simulink model "SVPWM_closeloop"  (R2022a)
settings: Solver=ode23t  StartTime=0.0  StopTime=1  RelTol=1e-3
InitFcn:
  | disp('开关频率20000Hz')
  | Ts = 1/20000;
libraries: spsIGBTDiodeLib x12, spsSeriesRLCBranchLib x11, spsDiodeLib x6, slpidlib x5, spsVoltageMeasurementLib x4, spsabctodq0Lib x3, spsThreePhaseVIMeasurementLib x2, spsDCVoltageSourceLib x1, spsGroundLib x1, spsPower3phInstantaneousLib x1, simulink x1, spsdq0toabcLib x1
settings Model: Creator=Ziang Liu  LastModifiedBy=Ziang Liu
settings DataIOCC: ReturnWorkspaceOutputs=off

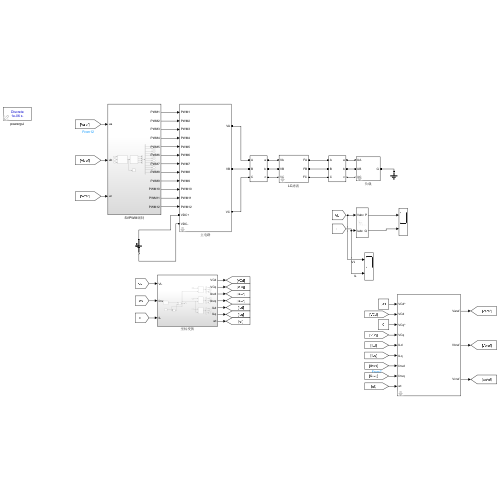
[thumbnail: Simulink's stored preview of the top-level diagram]
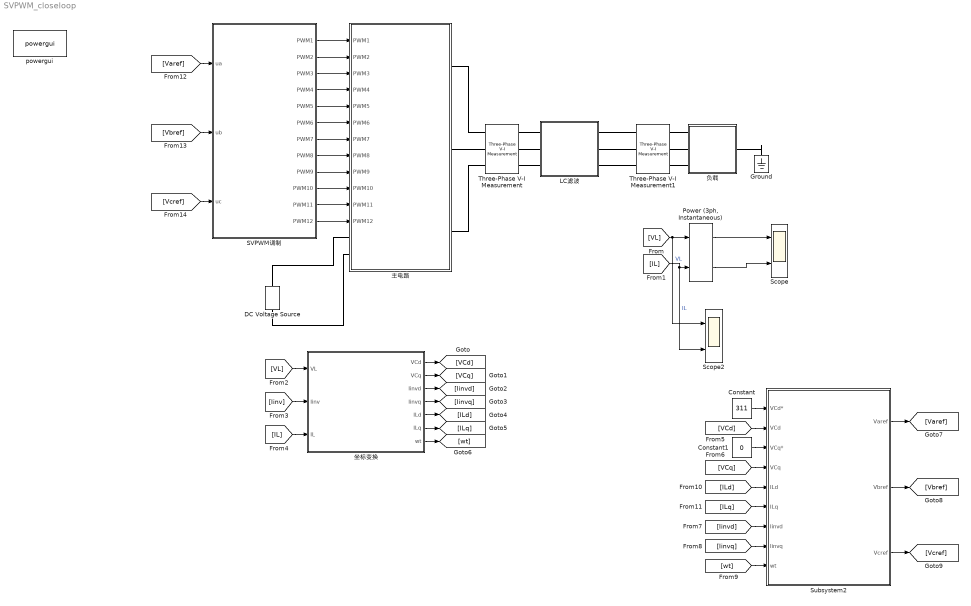
== system SVPWM_closeloop ==
  Constant : Constant  Value=311
  Constant1 : Constant  Value=0
  DC Voltage Source : spsDCVoltageSourceLib/DC Voltage Source  Amplitude=800  Measurements=None
  Ground : spsGroundLib/Ground  LConnTagsString=a
  LC滤波 : Subsystem  mask{L0=2e-3, R0=1e-3, Cf=10.5e-6, RC=3}
      mask prompts: L0 "滤波电感L0："; R0 "寄生电阻R0"; Cf "滤波电容Cf："; RC "无源阻尼RC："
      mask DialogControl ParameterGroupVar Prompt: 参数
  "Power (3ph, Instantaneous)" : spsPower3phInstantaneousLib/Power (3ph, Instantaneous)
  SVPWM调制 : Subsystem
  Scope : Scope  NumInputPorts=2
  Scope2 : Scope  NumInputPorts=2
  Subsystem2 : Subsystem  mask{Kp1=1.0825, Ki1=27.59, Kp2=13.3, Ki2=6.67, wC=2*pi*50*10.5e-6, wL=2*pi*50*2e-3}
      mask prompts: Kp1 "电压外环Kp1"; Ki1 "电压外环Ki1"; Kp2 "电流内环Kp2"; Ki2 "电流内环Ki2"; wC "电容耦合wC"; wL "电感耦合wL"
      mask DialogControl ParameterGroupVar Prompt: 参数
  Three-Phase V-I Measurement : spsThreePhaseVIMeasurementLib/Three-Phase V-I Measurement  VoltageMeasurement=no  SetLabelV=off  LabelV=Vabc  Vpu=off  VpuLL=off  CurrentMeasurement=yes  SetLabelI=on  LabelI=Iinv  Ipu=off  Pbase=100e6  Vbase=500e3  OutputType=Complex  PhasorSimulation=off  PSBequivalent=0
  Three-Phase V-I Measurement1 : spsThreePhaseVIMeasurementLib/Three-Phase V-I Measurement  VoltageMeasurement=phase-to-ground  SetLabelV=on  LabelV=VL  Vpu=off  VpuLL=off  CurrentMeasurement=yes  SetLabelI=on  LabelI=IL  Ipu=off  Pbase=100e6  Vbase=500e3  OutputType=Complex  PhasorSimulation=off  PSBequivalent=0
  powergui : spspowerguiLib/powergui  Priority=1  SimulationMode=Discrete  SampleTime=1e-6  frequency=60  Iterations=50  frequencyindice=0  Pbase=100e6  ErrMax=1e-4  UnitsV=kV  UnitsW=MW  buscounter=0  FunctionMessages=off  echomessages=off  EnableUseOfTLC=off  CurrentSourceSwitches=off  DisableSnubberDevices=off  DisableRonSwitches=off  DisableVfSwitches=off  DisplayEquations=off  AutomaticDiscreteSolvers=off  SolverType=Tustin/Backward Euler (TBE)  Interpol=off  ExternalGateDelay=off  methode=off  Ts=100  x0status=blocks  SPID=on  SwTol=0  HookPort=off  NonlinearTolerance=1e-4  nMaxIteration=100  ContinueOnMaxIteration=off  RestoreLinks=warning  ResistiveCurrentMeasurement=off  Frange=[0:2:500]  Ylog=off  Xlog=on  ShowGrid=off  save=off  variable=ZData  structure=0  ZoomFFT=off  StartTime=0.0  cycles=1  DisplayStyle=1  fundamental=60  FreqAxis=off  MaxFrequency=1000  frequencyindicesteady=1  RmsSteady=1  display=off
  主电路 : Subsystem  mask{C0=5600e-6}
      mask prompts: C0 "直流电容C0:"
      mask DialogControl ParameterGroupVar Prompt: 参数
  坐标变换 : Subsystem
  负载 : Subsystem  mask{R=1.44, L=0, C=3e-3}
      mask prompts: R "负载电阻R"; L "负载电感L"; C "负载电容C"
      mask DialogControl ParameterGroupVar Prompt: 参数
  wires:
  [Varef] -> SVPWM调制/1(ua)
  [Vbref] -> SVPWM调制/2(ub)
  [Vcref] -> SVPWM调制/3(uc)
  SVPWM调制/1(PWM1) -> 主电路/1(PWM1)
  SVPWM调制/2(PWM2) -> 主电路/2(PWM2)
  SVPWM调制/3(PWM3) -> 主电路/3(PWM3)
  SVPWM调制/4(PWM4) -> 主电路/4(PWM4)
  SVPWM调制/5(PWM5) -> 主电路/5(PWM5)
  SVPWM调制/6(PWM6) -> 主电路/6(PWM6)
  SVPWM调制/7(PWM7) -> 主电路/7(PWM7)
  SVPWM调制/8(PWM8) -> 主电路/8(PWM8)
  SVPWM调制/9(PWM9) -> 主电路/9(PWM9)
  SVPWM调制/10(PWM10) -> 主电路/10(PWM10)
  SVPWM调制/11(PWM11) -> 主电路/11(PWM11)
  SVPWM调制/12(PWM12) -> 主电路/12(PWM12)
  [VL] -> Scope2/1, "Power (3ph, Instantaneous)"/1  "VL"
  [IL] -> Scope2/2, "Power (3ph, Instantaneous)"/2  "IL"
  "Power (3ph, Instantaneous)"/1 -> Scope/1
  "Power (3ph, Instantaneous)"/2 -> Scope/2
  [Iinv] -> 坐标变换/2(Iinv)
  [VL] -> 坐标变换/1(VL)
  [IL] -> 坐标变换/3(IL)
  坐标变换/1(VCd) -> [VCd]
  坐标变换/2(VCq) -> [VCq]
  坐标变换/3(Iinvd) -> [Iinvd]
  坐标变换/4(Iinvq) -> [Iinvq]
  坐标变换/5(ILd) -> [ILd]
  坐标变换/6(ILq) -> [ILq]
  坐标变换/7(wt) -> [wt]
  Constant/1 -> Subsystem2/1(VCd*)
  Constant1/1 -> Subsystem2/3(VCq*)
  [VCd] -> Subsystem2/2(VCd)
  [VCq] -> Subsystem2/4(VCq)
  [Iinvd] -> Subsystem2/7(Iinvd)
  [Iinvq] -> Subsystem2/8(Iinvq)
  [wt] -> Subsystem2/9(wt)
  [ILd] -> Subsystem2/5(ILd)
  [ILq] -> Subsystem2/6(ILq)
  Subsystem2/1(Varef) -> [Varef]
  Subsystem2/2(Vbref) -> [Vbref]
  Subsystem2/3(Vcref) -> [Vcref]
  connections:
  DC Voltage Source/RConn1 -- 主电路/LConn1
  DC Voltage Source/LConn1 -- 主电路/LConn2
  Three-Phase V-I Measurement/LConn2 -- 主电路/RConn2
  主电路/RConn1 -- Three-Phase V-I Measurement/LConn1
  主电路/RConn3 -- Three-Phase V-I Measurement/LConn3
  LC滤波/LConn1 -- Three-Phase V-I Measurement/RConn1
  LC滤波/LConn2 -- Three-Phase V-I Measurement/RConn2
  LC滤波/LConn3 -- Three-Phase V-I Measurement/RConn3
  Three-Phase V-I Measurement1/LConn1 -- LC滤波/RConn1
  Three-Phase V-I Measurement1/LConn2 -- LC滤波/RConn2
  Three-Phase V-I Measurement1/LConn3 -- LC滤波/RConn3
  负载/LConn1 -- Three-Phase V-I Measurement1/RConn1
  负载/LConn2 -- Three-Phase V-I Measurement1/RConn2
  负载/LConn3 -- Three-Phase V-I Measurement1/RConn3
  Ground/LConn1 -- 负载/RConn1

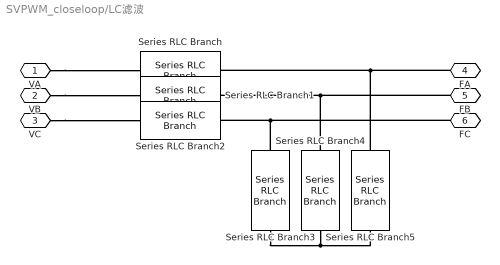
== system SVPWM_closeloop/LC滤波 ==
  Series RLC Branch : spsSeriesRLCBranchLib/Series RLC Branch  LConnTagsString=__new0  RConnTagsString=__new0  BranchType=RL  Resistance=R0  Inductance=L0  SetiL0=off  InitialCurrent=0  Capacitance=1e-6  Setx0=off  InitialVoltage=0  Measurements=None
  Series RLC Branch1 : spsSeriesRLCBranchLib/Series RLC Branch  LConnTagsString=__new0  RConnTagsString=__new0  BranchType=RL  Resistance=R0  Inductance=L0  SetiL0=off  InitialCurrent=0  Capacitance=1e-6  Setx0=off  InitialVoltage=0  Measurements=None
  Series RLC Branch2 : spsSeriesRLCBranchLib/Series RLC Branch  LConnTagsString=__new0  RConnTagsString=__new0  BranchType=RL  Resistance=R0  Inductance=L0  SetiL0=off  InitialCurrent=0  Capacitance=1e-6  Setx0=off  InitialVoltage=0  Measurements=None
  Series RLC Branch3 : spsSeriesRLCBranchLib/Series RLC Branch  LConnTagsString=__new0  RConnTagsString=__new0  BranchType=RC  Resistance=RC  Inductance=L0  SetiL0=off  InitialCurrent=0  Capacitance=Cf  Setx0=off  InitialVoltage=0  Measurements=None
  Series RLC Branch4 : spsSeriesRLCBranchLib/Series RLC Branch  LConnTagsString=__new0  RConnTagsString=__new0  BranchType=RC  Resistance=RC  Inductance=L0  SetiL0=off  InitialCurrent=0  Capacitance=Cf  Setx0=off  InitialVoltage=0  Measurements=None
  Series RLC Branch5 : spsSeriesRLCBranchLib/Series RLC Branch  LConnTagsString=__new0  RConnTagsString=__new0  BranchType=RC  Resistance=RC  Inductance=L0  SetiL0=off  InitialCurrent=0  Capacitance=Cf  Setx0=off  InitialVoltage=0  Measurements=None
  VA : PMIOPort  Side=Left
  VB : PMIOPort  Port=2  Side=Left
  VC : PMIOPort  Port=3  Side=Left
  FA : PMIOPort  Port=4  Side=Right
  FB : PMIOPort  Port=5  Side=Right
  FC : PMIOPort  Port=6  Side=Right
  connections:
  Series RLC Branch3/LConn1 -- FC/RConn1 -- Series RLC Branch2/RConn1
  Series RLC Branch4/LConn1 -- FB/RConn1 -- Series RLC Branch1/RConn1
  Series RLC Branch3/RConn1 -- Series RLC Branch4/RConn1 -- Series RLC Branch5/RConn1
  Series RLC Branch5/LConn1 -- FA/RConn1 -- Series RLC Branch/RConn1
  VB/RConn1 -- Series RLC Branch1/LConn1
  VA/RConn1 -- Series RLC Branch/LConn1
  VC/RConn1 -- Series RLC Branch2/LConn1

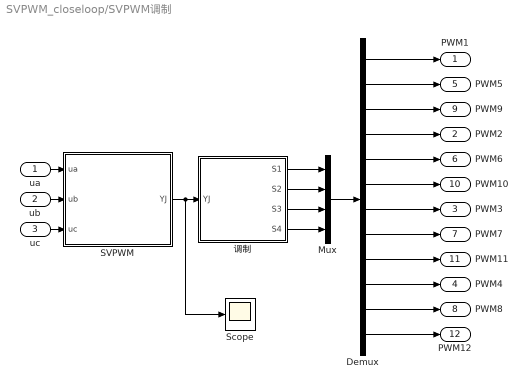
== system SVPWM_closeloop/SVPWM调制 ==
  ua : Inport
  ub : Inport  Port=2
  uc : Inport  Port=3
  Demux : Demux  Outputs=12
  Mux : Mux
  SVPWM : Subsystem
  Scope : Scope
  调制 : Subsystem
  PWM1 : Outport
  PWM2 : Outport  Port=2
  PWM3 : Outport  Port=3
  PWM4 : Outport  Port=4
  PWM5 : Outport  Port=5
  PWM6 : Outport  Port=6
  PWM7 : Outport  Port=7
  PWM8 : Outport  Port=8
  PWM9 : Outport  Port=9
  PWM10 : Outport  Port=10
  PWM11 : Outport  Port=11
  PWM12 : Outport  Port=12
  wires:
  Demux/4 -> PWM2/1
  Demux/9 -> PWM11/1
  SVPWM/1(YJ) -> Scope/1, 调制/1(YJ)
  ub/1 -> SVPWM/2(ub)
  Mux/1 -> Demux/1
  Demux/10 -> PWM4/1
  Demux/2 -> PWM5/1
  Demux/1 -> PWM1/1
  Demux/3 -> PWM9/1
  Demux/8 -> PWM7/1
  ua/1 -> SVPWM/1(ua)
  Demux/11 -> PWM8/1
  Demux/5 -> PWM6/1
  调制/4(S4) -> Mux/4
  调制/1(S1) -> Mux/1
  Demux/6 -> PWM10/1
  Demux/12 -> PWM12/1
  uc/1 -> SVPWM/3(uc)
  调制/3(S3) -> Mux/3
  调制/2(S2) -> Mux/2
  Demux/7 -> PWM3/1

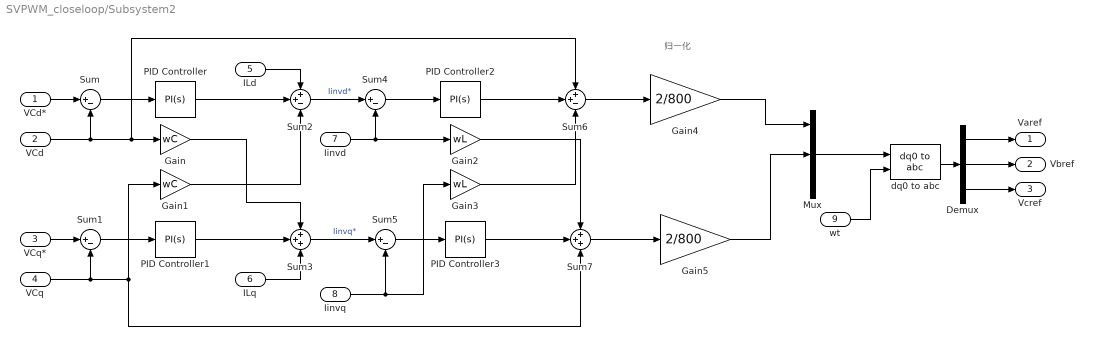
== system SVPWM_closeloop/Subsystem2 ==
  note: 归一化
  VCd* : Inport
  VCd : Inport  Port=2
  VCq* : Inport  Port=3
  VCq : Inport  Port=4
  ILd : Inport  Port=5
  ILq : Inport  Port=6
  Iinvd : Inport  Port=7
  Iinvq : Inport  Port=8
  wt : Inport  Port=9
  Demux : Demux  Outputs=3
  Gain : Gain  Gain=wC
  Gain1 : Gain  Gain=wC
  Gain2 : Gain  Gain=wL
  Gain3 : Gain  Gain=wL
  Gain4 : Gain  Gain=2/800
  Gain5 : Gain  Gain=2/800
  Mux : Mux  Inputs=3
  PID Controller : slpidlib/PID Controller  Controller=PI  Form=Parallel  TimeDomain=Continuous-time  UseExternalTs=off  SampleTime=-1  IntegratorMethod=Forward Euler  FilterMethod=Forward Euler  ControllerParametersSource=internal  P=Kp1  I=Ki1  UseKiTs=off  D=0  N=100  UseFilter=on  TunerSelectOption=Transfer Function Based (PID Tuner App)  InitialConditionSource=internal  InitialConditionForIntegrator=0  InitialConditionForFilter=0  DifferentiatorICPrevScaledInput=0  ExternalReset=none  TrackingMode=off  Kt=1  LimitOutput=off  SatLimitsSource=internal  UpperSaturationLimit=inf  LowerSaturationLimit=-inf  LinearizeAsGain=on  AntiWindupMode=none  Kb=1  POutMin=[]  POutMax=[]  IOutMin=[]  IOutMax=[]  DOutMin=[]  DOutMax=[]  NOutMin=[]  NOutMax=[]  SumOutMin=[]  SumOutMax=[]  SaturationOutMin=[]  SaturationOutMax=[]  PParamMin=[]  PParamMax=[]  IParamMin=[]  IParamMax=[]  DParamMin=[]  DParamMax=[]  NParamMin=[]  NParamMax=[]  KbParamMin=[]  KbParamMax=[]  KtParamMin=[]  KtParamMax=[]  KbOutMin=[]  KbOutMax=[]  KtOutMin=[]  KtOutMax=[]  IntegratorOutMin=[]  IntegratorOutMax=[]  FilterOutMin=[]  FilterOutMax=[]  SumI1OutMin=[]  SumI1OutMax=[]  SumI2OutMin=[]  SumI2OutMax=[]  SumI3OutMin=[]  SumI3OutMax=[]  SumI4OutMin=[]  SumI4OutMax=[]  SumDOutMin=[]  SumDOutMax=[]  DifferentiatorOutMin=[]  DifferentiatorOutMax=[]  FilterDiffOutCoefMin=[]  FilterDiffOutCoefMax=[]  ReciprocalOutMin=[]  ReciprocalOutMax=[]  SumDenOutMin=[]  SumDenOutMax=[]  SumNumOutMin=[]  SumNumOutMax=[]  DivideOutMin=[]  DivideOutMax=[]  UdiffTsProdOutMin=[]  UdiffTsProdOutMax=[]  NTsProdOutMin=[]  NTsProdOutMax=[]  UintegralTsProdOutMin=[]  UintegralTsProdOutMax=[]  UngainTsProdOutMin=[]  UngainTsProdOutMax=[]  IntegratorContinuousStateAttributes=''  IntegratorStateMustResolveToSignalObject=off  IntegratorRTWStateStorageClass=Auto  FilterContinuousStateAttributes=''  FilterStateMustResolveToSignalObject=off  FilterRTWStateStorageClass=Auto  ParallelPVariant=InternalParameters  IdealPVariant=Disabled  IVariant=InternalParameters  DVariant=Disabled  IntegratorVariant=Continuous  SatVariant=Disabled  AWVariant=Passthrough  PCopyVariant=Disabled  TRVariant=Disabled  FdbkBlocksVariant=Forward  IdealPFdbkVariant=Disabled  SatFdbkVariant=Disabled  DerivativeFilterVariant=Disabled  NVariant=Disabled  NCopyVariant=Disabled_SignalSpec  FilterICVariant=Disabled  IntegratorICVariant=InternalICs  ExternalResetVariant=Disabled  TRSumVariant=Passthrough  SumFdbkVariant=Disabled  SumVariant=Sum_PI  TsampFilterVariant=InternalTs  TsampNgainVariant=Passthrough  TsampIntegralVariant=Passthrough  ExternalSaturationOutDataTypeStr=Inherit: Same as second input  aMode=0
  PID Controller1 : slpidlib/PID Controller  Controller=PI  Form=Parallel  TimeDomain=Continuous-time  UseExternalTs=off  SampleTime=-1  IntegratorMethod=Forward Euler  FilterMethod=Forward Euler  ControllerParametersSource=internal  P=Kp1  I=Ki1  UseKiTs=off  D=0  N=100  UseFilter=on  TunerSelectOption=Transfer Function Based (PID Tuner App)  InitialConditionSource=internal  InitialConditionForIntegrator=0  InitialConditionForFilter=0  DifferentiatorICPrevScaledInput=0  ExternalReset=none  TrackingMode=off  Kt=1  LimitOutput=off  SatLimitsSource=internal  UpperSaturationLimit=inf  LowerSaturationLimit=-inf  LinearizeAsGain=on  AntiWindupMode=none  Kb=1  POutMin=[]  POutMax=[]  IOutMin=[]  IOutMax=[]  DOutMin=[]  DOutMax=[]  NOutMin=[]  NOutMax=[]  SumOutMin=[]  SumOutMax=[]  SaturationOutMin=[]  SaturationOutMax=[]  PParamMin=[]  PParamMax=[]  IParamMin=[]  IParamMax=[]  DParamMin=[]  DParamMax=[]  NParamMin=[]  NParamMax=[]  KbParamMin=[]  KbParamMax=[]  KtParamMin=[]  KtParamMax=[]  KbOutMin=[]  KbOutMax=[]  KtOutMin=[]  KtOutMax=[]  IntegratorOutMin=[]  IntegratorOutMax=[]  FilterOutMin=[]  FilterOutMax=[]  SumI1OutMin=[]  SumI1OutMax=[]  SumI2OutMin=[]  SumI2OutMax=[]  SumI3OutMin=[]  SumI3OutMax=[]  SumI4OutMin=[]  SumI4OutMax=[]  SumDOutMin=[]  SumDOutMax=[]  DifferentiatorOutMin=[]  DifferentiatorOutMax=[]  FilterDiffOutCoefMin=[]  FilterDiffOutCoefMax=[]  ReciprocalOutMin=[]  ReciprocalOutMax=[]  SumDenOutMin=[]  SumDenOutMax=[]  SumNumOutMin=[]  SumNumOutMax=[]  DivideOutMin=[]  DivideOutMax=[]  UdiffTsProdOutMin=[]  UdiffTsProdOutMax=[]  NTsProdOutMin=[]  NTsProdOutMax=[]  UintegralTsProdOutMin=[]  UintegralTsProdOutMax=[]  UngainTsProdOutMin=[]  UngainTsProdOutMax=[]  IntegratorContinuousStateAttributes=''  IntegratorStateMustResolveToSignalObject=off  IntegratorRTWStateStorageClass=Auto  FilterContinuousStateAttributes=''  FilterStateMustResolveToSignalObject=off  FilterRTWStateStorageClass=Auto  ParallelPVariant=InternalParameters  IdealPVariant=Disabled  IVariant=InternalParameters  DVariant=Disabled  IntegratorVariant=Continuous  SatVariant=Disabled  AWVariant=Passthrough  PCopyVariant=Disabled  TRVariant=Disabled  FdbkBlocksVariant=Forward  IdealPFdbkVariant=Disabled  SatFdbkVariant=Disabled  DerivativeFilterVariant=Disabled  NVariant=Disabled  NCopyVariant=Disabled_SignalSpec  FilterICVariant=Disabled  IntegratorICVariant=InternalICs  ExternalResetVariant=Disabled  TRSumVariant=Passthrough  SumFdbkVariant=Disabled  SumVariant=Sum_PI  TsampFilterVariant=InternalTs  TsampNgainVariant=Passthrough  TsampIntegralVariant=Passthrough  ExternalSaturationOutDataTypeStr=Inherit: Same as second input  aMode=0
  PID Controller2 : slpidlib/PID Controller  Controller=PI  Form=Parallel  TimeDomain=Continuous-time  UseExternalTs=off  SampleTime=-1  IntegratorMethod=Forward Euler  FilterMethod=Forward Euler  ControllerParametersSource=internal  P=Kp2  I=Ki2  UseKiTs=off  D=0  N=100  UseFilter=on  TunerSelectOption=Transfer Function Based (PID Tuner App)  InitialConditionSource=internal  InitialConditionForIntegrator=0  InitialConditionForFilter=0  DifferentiatorICPrevScaledInput=0  ExternalReset=none  TrackingMode=off  Kt=1  LimitOutput=off  SatLimitsSource=internal  UpperSaturationLimit=inf  LowerSaturationLimit=-inf  LinearizeAsGain=on  AntiWindupMode=none  Kb=1  POutMin=[]  POutMax=[]  IOutMin=[]  IOutMax=[]  DOutMin=[]  DOutMax=[]  NOutMin=[]  NOutMax=[]  SumOutMin=[]  SumOutMax=[]  SaturationOutMin=[]  SaturationOutMax=[]  PParamMin=[]  PParamMax=[]  IParamMin=[]  IParamMax=[]  DParamMin=[]  DParamMax=[]  NParamMin=[]  NParamMax=[]  KbParamMin=[]  KbParamMax=[]  KtParamMin=[]  KtParamMax=[]  KbOutMin=[]  KbOutMax=[]  KtOutMin=[]  KtOutMax=[]  IntegratorOutMin=[]  IntegratorOutMax=[]  FilterOutMin=[]  FilterOutMax=[]  SumI1OutMin=[]  SumI1OutMax=[]  SumI2OutMin=[]  SumI2OutMax=[]  SumI3OutMin=[]  SumI3OutMax=[]  SumI4OutMin=[]  SumI4OutMax=[]  SumDOutMin=[]  SumDOutMax=[]  DifferentiatorOutMin=[]  DifferentiatorOutMax=[]  FilterDiffOutCoefMin=[]  FilterDiffOutCoefMax=[]  ReciprocalOutMin=[]  ReciprocalOutMax=[]  SumDenOutMin=[]  SumDenOutMax=[]  SumNumOutMin=[]  SumNumOutMax=[]  DivideOutMin=[]  DivideOutMax=[]  UdiffTsProdOutMin=[]  UdiffTsProdOutMax=[]  NTsProdOutMin=[]  NTsProdOutMax=[]  UintegralTsProdOutMin=[]  UintegralTsProdOutMax=[]  UngainTsProdOutMin=[]  UngainTsProdOutMax=[]  IntegratorContinuousStateAttributes=''  IntegratorStateMustResolveToSignalObject=off  IntegratorRTWStateStorageClass=Auto  FilterContinuousStateAttributes=''  FilterStateMustResolveToSignalObject=off  FilterRTWStateStorageClass=Auto  ParallelPVariant=InternalParameters  IdealPVariant=Disabled  IVariant=InternalParameters  DVariant=Disabled  IntegratorVariant=Continuous  SatVariant=Disabled  AWVariant=Passthrough  PCopyVariant=Disabled  TRVariant=Disabled  FdbkBlocksVariant=Forward  IdealPFdbkVariant=Disabled  SatFdbkVariant=Disabled  DerivativeFilterVariant=Disabled  NVariant=Disabled  NCopyVariant=Disabled_SignalSpec  FilterICVariant=Disabled  IntegratorICVariant=InternalICs  ExternalResetVariant=Disabled  TRSumVariant=Passthrough  SumFdbkVariant=Disabled  SumVariant=Sum_PI  TsampFilterVariant=InternalTs  TsampNgainVariant=Passthrough  TsampIntegralVariant=Passthrough  ExternalSaturationOutDataTypeStr=Inherit: Same as second input  aMode=0
  PID Controller3 : slpidlib/PID Controller  Controller=PI  Form=Parallel  TimeDomain=Continuous-time  UseExternalTs=off  SampleTime=-1  IntegratorMethod=Forward Euler  FilterMethod=Forward Euler  ControllerParametersSource=internal  P=Kp2  I=Ki2  UseKiTs=off  D=0  N=100  UseFilter=on  TunerSelectOption=Transfer Function Based (PID Tuner App)  InitialConditionSource=internal  InitialConditionForIntegrator=0  InitialConditionForFilter=0  DifferentiatorICPrevScaledInput=0  ExternalReset=none  TrackingMode=off  Kt=1  LimitOutput=off  SatLimitsSource=internal  UpperSaturationLimit=inf  LowerSaturationLimit=-inf  LinearizeAsGain=on  AntiWindupMode=none  Kb=1  POutMin=[]  POutMax=[]  IOutMin=[]  IOutMax=[]  DOutMin=[]  DOutMax=[]  NOutMin=[]  NOutMax=[]  SumOutMin=[]  SumOutMax=[]  SaturationOutMin=[]  SaturationOutMax=[]  PParamMin=[]  PParamMax=[]  IParamMin=[]  IParamMax=[]  DParamMin=[]  DParamMax=[]  NParamMin=[]  NParamMax=[]  KbParamMin=[]  KbParamMax=[]  KtParamMin=[]  KtParamMax=[]  KbOutMin=[]  KbOutMax=[]  KtOutMin=[]  KtOutMax=[]  IntegratorOutMin=[]  IntegratorOutMax=[]  FilterOutMin=[]  FilterOutMax=[]  SumI1OutMin=[]  SumI1OutMax=[]  SumI2OutMin=[]  SumI2OutMax=[]  SumI3OutMin=[]  SumI3OutMax=[]  SumI4OutMin=[]  SumI4OutMax=[]  SumDOutMin=[]  SumDOutMax=[]  DifferentiatorOutMin=[]  DifferentiatorOutMax=[]  FilterDiffOutCoefMin=[]  FilterDiffOutCoefMax=[]  ReciprocalOutMin=[]  ReciprocalOutMax=[]  SumDenOutMin=[]  SumDenOutMax=[]  SumNumOutMin=[]  SumNumOutMax=[]  DivideOutMin=[]  DivideOutMax=[]  UdiffTsProdOutMin=[]  UdiffTsProdOutMax=[]  NTsProdOutMin=[]  NTsProdOutMax=[]  UintegralTsProdOutMin=[]  UintegralTsProdOutMax=[]  UngainTsProdOutMin=[]  UngainTsProdOutMax=[]  IntegratorContinuousStateAttributes=''  IntegratorStateMustResolveToSignalObject=off  IntegratorRTWStateStorageClass=Auto  FilterContinuousStateAttributes=''  FilterStateMustResolveToSignalObject=off  FilterRTWStateStorageClass=Auto  ParallelPVariant=InternalParameters  IdealPVariant=Disabled  IVariant=InternalParameters  DVariant=Disabled  IntegratorVariant=Continuous  SatVariant=Disabled  AWVariant=Passthrough  PCopyVariant=Disabled  TRVariant=Disabled  FdbkBlocksVariant=Forward  IdealPFdbkVariant=Disabled  SatFdbkVariant=Disabled  DerivativeFilterVariant=Disabled  NVariant=Disabled  NCopyVariant=Disabled_SignalSpec  FilterICVariant=Disabled  IntegratorICVariant=InternalICs  ExternalResetVariant=Disabled  TRSumVariant=Passthrough  SumFdbkVariant=Disabled  SumVariant=Sum_PI  TsampFilterVariant=InternalTs  TsampNgainVariant=Passthrough  TsampIntegralVariant=Passthrough  ExternalSaturationOutDataTypeStr=Inherit: Same as second input  aMode=0
  Sum{,1,4..5} (4 alike) : Sum  Inputs=|+-
  Sum2 : Sum  Inputs=++-
  Sum3 : Sum  Inputs=+++
  Sum6 : Sum  Inputs=++-
  Sum7 : Sum  Inputs=+++
  dq0 to abc : spsdq0toabcLib/dq0 to abc  Alignment=90 degrees behind phase A axis
  Varef : Outport
  Vbref : Outport  Port=2
  Vcref : Outport  Port=3
  wires:
  Demux/2 -> Vbref/1
  Iinvd/1 -> Gain2/1, Sum4/2
  Demux/1 -> Varef/1
  Sum1/1 -> PID Controller1/1
  Gain2/1 -> Sum7/1
  VCd/1 -> Sum/2, Sum6/1, Gain/1
  Gain4/1 -> Mux/1
  VCq/1 -> Gain1/1, Sum7/3, Sum1/2
  Demux/3 -> Vcref/1
  Gain5/1 -> Mux/2
  wt/1 -> dq0 to abc/2
  Iinvq/1 -> Sum5/2, Gain3/1
  Sum4/1 -> PID Controller2/1
  ILd/1 -> Sum2/1
  ILq/1 -> Sum3/3
  Sum2/1 -> Sum4/1  "Iinvd*"
  Sum3/1 -> Sum5/1  "Iinvq*"
  Mux/1 -> dq0 to abc/1
  Gain1/1 -> Sum2/3
  Gain3/1 -> Sum6/3
  dq0 to abc/1 -> Demux/1
  PID Controller3/1 -> Sum7/2
  VCq*/1 -> Sum1/1
  PID Controller/1 -> Sum2/2
  Sum5/1 -> PID Controller3/1
  PID Controller1/1 -> Sum3/2
  Gain/1 -> Sum3/1
  PID Controller2/1 -> Sum6/2
  Sum/1 -> PID Controller/1
  Sum7/1 -> Gain5/1
  Sum6/1 -> Gain4/1
  VCd*/1 -> Sum/1

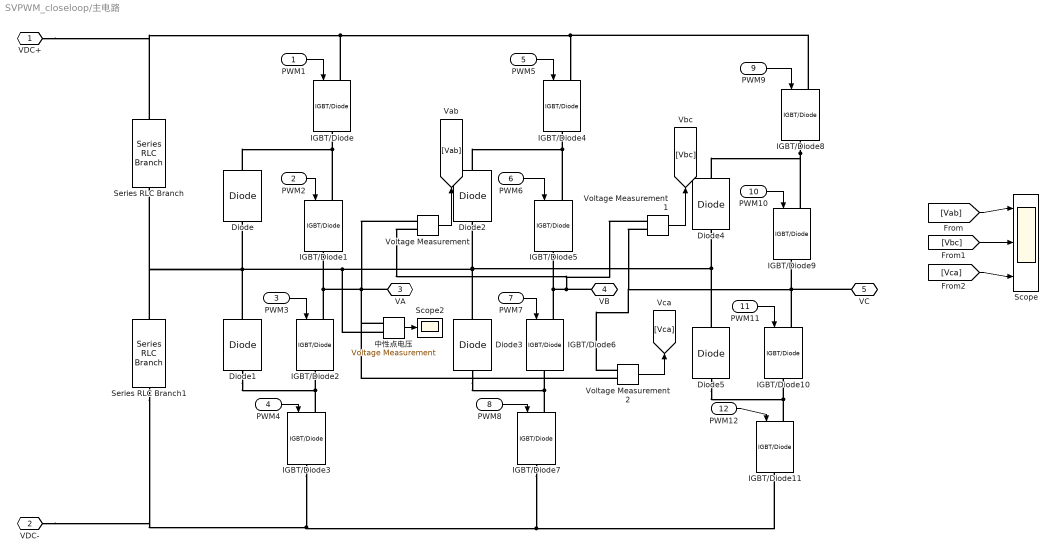
== system SVPWM_closeloop/主电路 ==
  PWM1 : Inport
  PWM2 : Inport  Port=2
  PWM3 : Inport  Port=3
  PWM4 : Inport  Port=4
  PWM5 : Inport  Port=5
  PWM6 : Inport  Port=6
  PWM7 : Inport  Port=7
  PWM8 : Inport  Port=8
  PWM9 : Inport  Port=9
  PWM10 : Inport  Port=10
  PWM11 : Inport  Port=11
  PWM12 : Inport  Port=12
  Diode{,1..5} (6 alike) : spsDiodeLib/Diode  Ron=0.001  Lon=0  Vf=0.8  IC=0  UseSnubber=0  Rs=500  Cs=250e-9  Measurements=off
  IGBT/Diode{,1..11} (12 alike) : spsIGBTDiodeLib/IGBT//Diode  Ron=1e-3  Rs=1e5  Cs=inf  Measurements=off
  Scope : Scope  NumInputPorts=3
  Scope2 : Scope
  Series RLC Branch : spsSeriesRLCBranchLib/Series RLC Branch  LConnTagsString=__new0  RConnTagsString=__new0  BranchType=RC  Resistance=1e-3  Inductance=1e-3  SetiL0=off  InitialCurrent=0  Capacitance=C0  Setx0=off  InitialVoltage=0  Measurements=None
  Series RLC Branch1 : spsSeriesRLCBranchLib/Series RLC Branch  LConnTagsString=__new0  RConnTagsString=__new0  BranchType=RC  Resistance=1e-3  Inductance=1e-3  SetiL0=off  InitialCurrent=0  Capacitance=C0  Setx0=off  InitialVoltage=0  Measurements=None
  Voltage Measurement : spsVoltageMeasurementLib/Voltage Measurement  PhasorSimulation=off  OutputType=Complex  PSBequivalent=0
  Voltage Measurement1 : spsVoltageMeasurementLib/Voltage Measurement  PhasorSimulation=off  OutputType=Complex  PSBequivalent=0
  Voltage Measurement2 : spsVoltageMeasurementLib/Voltage Measurement  PhasorSimulation=off  OutputType=Complex  PSBequivalent=0
  中性点电压 : spsVoltageMeasurementLib/Voltage Measurement  PhasorSimulation=off  OutputType=Complex  PSBequivalent=0
  VDC+ : PMIOPort  Side=Left
  VDC- : PMIOPort  Port=2  Side=Left
  VA : PMIOPort  Port=3  Side=Right
  VB : PMIOPort  Port=4  Side=Right
  VC : PMIOPort  Port=5  Side=Right
  wires:
  PWM8/1 -> IGBT/Diode7/1
  Voltage Measurement1/1 -> [Vbc]
  [Vbc] -> Scope/2
  PWM7/1 -> IGBT/Diode6/1
  PWM6/1 -> IGBT/Diode5/1
  PWM12/1 -> IGBT/Diode11/1
  PWM10/1 -> IGBT/Diode9/1
  PWM9/1 -> IGBT/Diode8/1
  PWM5/1 -> IGBT/Diode4/1
  PWM11/1 -> IGBT/Diode10/1
  PWM2/1 -> IGBT/Diode1/1
  中性点电压/1 -> Scope2/1
  PWM3/1 -> IGBT/Diode2/1
  Voltage Measurement2/1 -> [Vca]
  Voltage Measurement/1 -> [Vab]
  PWM1/1 -> IGBT/Diode/1
  PWM4/1 -> IGBT/Diode3/1
  [Vab] -> Scope/1
  [Vca] -> Scope/3
  connections:
  IGBT/Diode/LConn1 -- VDC+/RConn1 -- Series RLC Branch/LConn1 -- IGBT/Diode4/LConn1 -- IGBT/Diode8/LConn1
  IGBT/Diode3/RConn1 -- VDC-/RConn1 -- Series RLC Branch1/RConn1 -- IGBT/Diode7/RConn1 -- IGBT/Diode11/RConn1
  IGBT/Diode6/LConn1 -- VB/RConn1 -- Voltage Measurement1/LConn1 -- Voltage Measurement/LConn2 -- IGBT/Diode5/RConn1
  Diode3/RConn1 -- Diode4/LConn1 -- Diode5/RConn1 -- Diode2/LConn1 -- 中性点电压/LConn2 -- Series RLC Branch/RConn1 -- Series RLC Branch1/LConn1 -- Diode/LConn1 -- Diode1/RConn1
  IGBT/Diode10/LConn1 -- VC/RConn1 -- Voltage Measurement2/LConn1 -- Voltage Measurement1/LConn2 -- IGBT/Diode9/RConn1
  IGBT/Diode2/LConn1 -- VA/RConn1 -- 中性点电压/LConn1 -- Voltage Measurement2/LConn2 -- Voltage Measurement/LConn1 -- IGBT/Diode1/RConn1
  Diode3/LConn1 -- IGBT/Diode7/LConn1 -- IGBT/Diode6/RConn1
  IGBT/Diode1/LConn1 -- Diode/RConn1 -- IGBT/Diode/RConn1
  IGBT/Diode5/LConn1 -- IGBT/Diode4/RConn1 -- Diode2/RConn1
  IGBT/Diode3/LConn1 -- Diode1/LConn1 -- IGBT/Diode2/RConn1
  IGBT/Diode8/RConn1 -- IGBT/Diode9/LConn1 -- Diode4/RConn1
  IGBT/Diode11/LConn1 -- Diode5/LConn1 -- IGBT/Diode10/RConn1

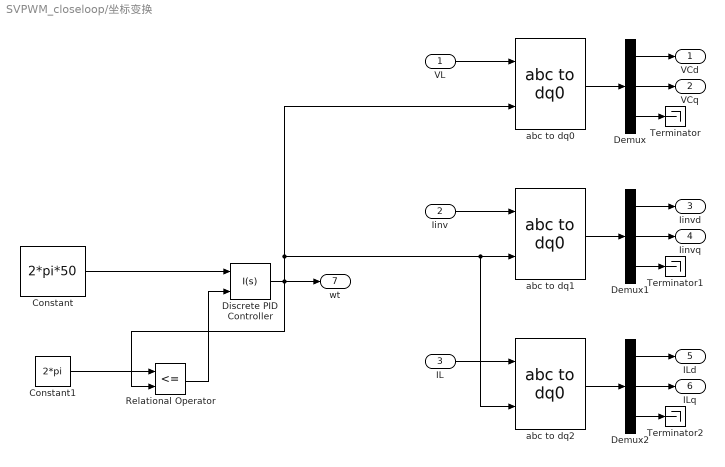
== system SVPWM_closeloop/坐标变换 ==
  VL : Inport
  Iinv : Inport  Port=2
  IL : Inport  Port=3
  Constant : Constant  Value=2*pi*50
  Constant1 : Constant  Value=2*pi
  Demux : Demux  Outputs=3
  Demux1 : Demux  Outputs=3
  Demux2 : Demux  Outputs=3
  Discrete PID Controller : slpidlib/PID Controller  Controller=I  Form=Parallel  TimeDomain=Continuous-time  UseExternalTs=off  SampleTime=-1  IntegratorMethod=Forward Euler  FilterMethod=Forward Euler  ControllerParametersSource=internal  P=1  I=1  UseKiTs=off  D=0  N=100  UseFilter=on  TunerSelectOption=Transfer Function Based (PID Tuner App)  ZeroCross=off  InitialConditionSource=internal  InitialConditionForIntegrator=0  InitialConditionForFilter=0  DifferentiatorICPrevScaledInput=0  ExternalReset=rising  TrackingMode=off  Kt=1  LimitOutput=off  SatLimitsSource=internal  UpperSaturationLimit=inf  LowerSaturationLimit=-inf  LinearizeAsGain=off  AntiWindupMode=none  Kb=1  POutMin=[]  POutMax=[]  IOutMin=[]  IOutMax=[]  DOutMin=[]  DOutMax=[]  NOutMin=[]  NOutMax=[]  SumOutMin=[]  SumOutMax=[]  SaturationOutMin=[]  SaturationOutMax=[]  PParamMin=[]  PParamMax=[]  IParamMin=[]  IParamMax=[]  DParamMin=[]  DParamMax=[]  NParamMin=[]  NParamMax=[]  KbParamMin=[]  KbParamMax=[]  KtParamMin=[]  KtParamMax=[]  KbOutMin=[]  KbOutMax=[]  KtOutMin=[]  KtOutMax=[]  IntegratorOutMin=[]  IntegratorOutMax=[]  FilterOutMin=[]  FilterOutMax=[]  SumI1OutMin=[]  SumI1OutMax=[]  SumI2OutMin=[]  SumI2OutMax=[]  SumI3OutMin=[]  SumI3OutMax=[]  SumI4OutMin=[]  SumI4OutMax=[]  SumDOutMin=[]  SumDOutMax=[]  DifferentiatorOutMin=[]  DifferentiatorOutMax=[]  FilterDiffOutCoefMin=[]  FilterDiffOutCoefMax=[]  ReciprocalOutMin=[]  ReciprocalOutMax=[]  SumDenOutMin=[]  SumDenOutMax=[]  SumNumOutMin=[]  SumNumOutMax=[]  DivideOutMin=[]  DivideOutMax=[]  UdiffTsProdOutMin=[]  UdiffTsProdOutMax=[]  NTsProdOutMin=[]  NTsProdOutMax=[]  UintegralTsProdOutMin=[]  UintegralTsProdOutMax=[]  UngainTsProdOutMin=[]  UngainTsProdOutMax=[]  IntegratorContinuousStateAttributes=''  IntegratorStateMustResolveToSignalObject=off  IntegratorRTWStateStorageClass=Auto  FilterContinuousStateAttributes=''  FilterStateMustResolveToSignalObject=off  FilterRTWStateStorageClass=Auto  ParallelPVariant=Disabled  IdealPVariant=Disabled  IVariant=InternalParameters  DVariant=Disabled  IntegratorVariant=Continuous  SatVariant=Disabled  AWVariant=Passthrough  PCopyVariant=Disabled  TRVariant=Disabled  FdbkBlocksVariant=Forward  IdealPFdbkVariant=Disabled  SatFdbkVariant=Disabled  DerivativeFilterVariant=Disabled  NVariant=Disabled  NCopyVariant=Disabled_SignalSpec  FilterICVariant=Disabled  IntegratorICVariant=InternalICs  ExternalResetVariant=ExternalReset  TRSumVariant=Passthrough  SumFdbkVariant=Disabled  SumVariant=Passthrough_I  TsampFilterVariant=InternalTs  TsampNgainVariant=Passthrough  TsampIntegralVariant=Passthrough  ExternalSaturationOutDataTypeStr=Inherit: Same as second input  aMode=0
  Relational Operator : RelationalOperator  Operator=<=  OutDataTypeStr=boolean  RndMeth=Simplest  InputSameDT=off
  Terminator : Terminator
  Terminator1 : Terminator
  Terminator2 : Terminator
  abc to dq0 : spsabctodq0Lib/abc to dq0  Alignment=90 degrees behind phase A axis
  abc to dq1 : spsabctodq0Lib/abc to dq0  Alignment=90 degrees behind phase A axis
  abc to dq2 : spsabctodq0Lib/abc to dq0  Alignment=90 degrees behind phase A axis
  VCd : Outport
  VCq : Outport  Port=2
  Iinvd : Outport  Port=3
  Iinvq : Outport  Port=4
  ILd : Outport  Port=5
  ILq : Outport  Port=6
  wt : Outport  Port=7
  wires:
  abc to dq2/1 -> Demux2/1
  Demux1/2 -> Iinvq/1
  Demux1/1 -> Iinvd/1
  Discrete PID Controller/1 -> wt/1, abc to dq2/2, abc to dq1/2, abc to dq0/2, Relational Operator/2
  Demux/3 -> Terminator/1
  Demux1/3 -> Terminator1/1
  Constant1/1 -> Relational Operator/1
  Demux/1 -> VCd/1
  Demux/2 -> VCq/1
  abc to dq1/1 -> Demux1/1
  Iinv/1 -> abc to dq1/1
  Relational Operator/1 -> Discrete PID Controller/2
  Constant/1 -> Discrete PID Controller/1
  abc to dq0/1 -> Demux/1
  VL/1 -> abc to dq0/1
  IL/1 -> abc to dq2/1
  Demux2/2 -> ILq/1
  Demux2/3 -> Terminator2/1
  Demux2/1 -> ILd/1

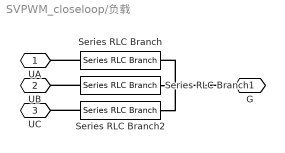
== system SVPWM_closeloop/负载 ==
  Series RLC Branch : spsSeriesRLCBranchLib/Series RLC Branch  LConnTagsString=__new0  RConnTagsString=__new0  BranchType=RLC  Resistance=R  Inductance=L  SetiL0=off  InitialCurrent=0  Capacitance=C  Setx0=off  InitialVoltage=0  Measurements=None
  Series RLC Branch1 : spsSeriesRLCBranchLib/Series RLC Branch  LConnTagsString=__new0  RConnTagsString=__new0  BranchType=RLC  Resistance=R  Inductance=L  SetiL0=off  InitialCurrent=0  Capacitance=C  Setx0=off  InitialVoltage=0  Measurements=None
  Series RLC Branch2 : spsSeriesRLCBranchLib/Series RLC Branch  LConnTagsString=__new0  RConnTagsString=__new0  BranchType=RLC  Resistance=R  Inductance=L  SetiL0=off  InitialCurrent=0  Capacitance=C  Setx0=off  InitialVoltage=0  Measurements=None
  UA : PMIOPort  Side=Left
  UB : PMIOPort  Port=2  Side=Left
  UC : PMIOPort  Port=3  Side=Left
  G : PMIOPort  Port=4  Side=Right
  connections:
  Series RLC Branch2/RConn1 -- G/RConn1 -- Series RLC Branch1/RConn1 -- Series RLC Branch/RConn1
  Series RLC Branch2/LConn1 -- UC/RConn1
  Series RLC Branch1/LConn1 -- UB/RConn1
  Series RLC Branch/LConn1 -- UA/RConn1

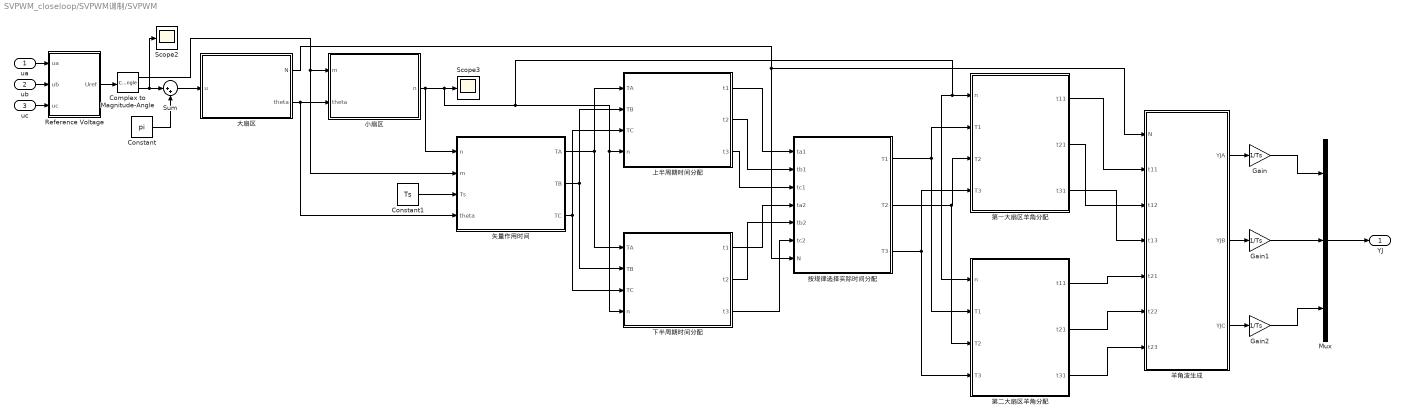
== system SVPWM_closeloop/SVPWM调制/SVPWM ==
  ua : Inport
  ub : Inport  Port=2
  uc : Inport  Port=3
  Complex to Magnitude-Angle : ComplexToMagnitudeAngle
  Constant : Constant  Value=pi
  Constant1 : Constant  Value=Ts
  Gain : Gain  Gain=1/Ts
  Gain1 : Gain  Gain=1/Ts
  Gain2 : Gain  Gain=1/Ts
  Mux : Mux  Inputs=3
  Reference Voltage : MATLAB Function  TreatAsAtomicUnit=on
  Scope2 : Scope
  Scope3 : Scope
  Sum : Sum  Inputs=|++
  上半周期时间分配 : MATLAB Function  TreatAsAtomicUnit=on
  下半周期时间分配 : MATLAB Function  TreatAsAtomicUnit=on
  大扇区 : MATLAB Function  TreatAsAtomicUnit=on
  小扇区 : MATLAB Function  TreatAsAtomicUnit=on
  按规律选择实际时间分配 : MATLAB Function  TreatAsAtomicUnit=on
  矢量作用时间 : MATLAB Function  TreatAsAtomicUnit=on
  第一大扇区羊角分配 : MATLAB Function  TreatAsAtomicUnit=on
  第二大扇区羊角分配 : MATLAB Function  TreatAsAtomicUnit=on
  羊角波生成 : MATLAB Function  TreatAsAtomicUnit=on
  YJ : Outport
  wires:
  按规律选择实际时间分配/1(T1) -> 第二大扇区羊角分配/2(T1), 第一大扇区羊角分配/2(T1)
  Constant1/1 -> 矢量作用时间/3(Ts)
  Gain/1 -> Mux/1
  Sum/1 -> 大扇区/1(u)
  矢量作用时间/2(TB) -> 上半周期时间分配/2(TB), 下半周期时间分配/2(TB)
  按规律选择实际时间分配/3(T3) -> 第二大扇区羊角分配/4(T3), 第一大扇区羊角分配/4(T3)
  矢量作用时间/3(TC) -> 上半周期时间分配/3(TC), 下半周期时间分配/3(TC)
  小扇区/1(n) -> 第一大扇区羊角分配/1(n), 第二大扇区羊角分配/1(n), 下半周期时间分配/4(n), 上半周期时间分配/4(n), Scope3/1, 矢量作用时间/1(n)
  Reference Voltage/1(Uref) -> Complex to Magnitude-Angle/1
  Gain1/1 -> Mux/2
  上半周期时间分配/3(t3) -> 按规律选择实际时间分配/3(tc1)
  下半周期时间分配/2(t2) -> 按规律选择实际时间分配/5(tb2)
  下半周期时间分配/1(t1) -> 按规律选择实际时间分配/4(ta2)
  大扇区/1(N) -> 按规律选择实际时间分配/7(N), 羊角波生成/1(N)
  Constant/1 -> Sum/2
  上半周期时间分配/2(t2) -> 按规律选择实际时间分配/2(tb1)
  第二大扇区羊角分配/2(t21) -> 羊角波生成/6(t22)
  Complex to Magnitude-Angle/1 -> 矢量作用时间/2(m), 小扇区/1(m)
  大扇区/2(theta) -> 小扇区/2(theta), 矢量作用时间/4(theta)
  第一大扇区羊角分配/2(t21) -> 羊角波生成/3(t12)
  第一大扇区羊角分配/3(t31) -> 羊角波生成/4(t13)
  下半周期时间分配/3(t3) -> 按规律选择实际时间分配/6(tc2)
  第二大扇区羊角分配/1(t11) -> 羊角波生成/5(t21)
  ub/1 -> Reference Voltage/2(ub)
  Complex to Magnitude-Angle/2 -> Scope2/1, Sum/1
  羊角波生成/1(YJA) -> Gain/1
  第一大扇区羊角分配/1(t11) -> 羊角波生成/2(t11)
  上半周期时间分配/1(t1) -> 按规律选择实际时间分配/1(ta1)
  矢量作用时间/1(TA) -> 下半周期时间分配/1(TA), 上半周期时间分配/1(TA)
  羊角波生成/2(YJB) -> Gain1/1
  按规律选择实际时间分配/2(T2) -> 第二大扇区羊角分配/3(T2), 第一大扇区羊角分配/3(T2)
  羊角波生成/3(YJC) -> Gain2/1
  第二大扇区羊角分配/3(t31) -> 羊角波生成/7(t23)
  ua/1 -> Reference Voltage/1(ua)
  Mux/1 -> YJ/1
  Gain2/1 -> Mux/3
  uc/1 -> Reference Voltage/3(uc)

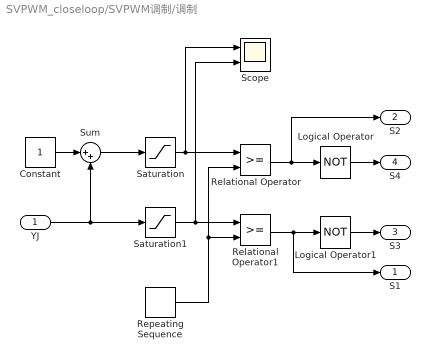
== system SVPWM_closeloop/SVPWM调制/调制 ==
  YJ : Inport
  Constant : Constant
  Logical Operator : Logic  Operator=NOT  AllPortsSameDT=off  OutDataTypeStr=boolean
  Logical Operator1 : Logic  Operator=NOT  AllPortsSameDT=off  OutDataTypeStr=boolean
  Relational Operator : RelationalOperator  OutDataTypeStr=boolean  RndMeth=Simplest  InputSameDT=off
  Relational Operator1 : RelationalOperator  OutDataTypeStr=boolean  RndMeth=Simplest  InputSameDT=off
  Repeating Sequence : simulink/Sources/Repeating Sequence  rep_seq_t=[0 0.5*Ts Ts]  rep_seq_y=[1 0 1]
  Saturation : Saturate  UpperLimit=1  LowerLimit=0
  Saturation1 : Saturate  UpperLimit=1  LowerLimit=0
  Scope : Scope  NumInputPorts=2
  Sum : Sum  Inputs=|++
  S1 : Outport
  S2 : Outport  Port=2
  S3 : Outport  Port=3
  S4 : Outport  Port=4
  wires:
  Constant/1 -> Sum/1
  Relational Operator1/1 -> S1/1, Logical Operator1/1
  Saturation/1 -> Scope/1, Relational Operator/1
  YJ/1 -> Saturation1/1, Sum/2
  Relational Operator/1 -> S2/1, Logical Operator/1
  Logical Operator/1 -> S4/1
  Logical Operator1/1 -> S3/1
  Sum/1 -> Saturation/1
  Repeating Sequence/1 -> Relational Operator1/2, Relational Operator/2
  Saturation1/1 -> Scope/2, Relational Operator1/1

== matlab function SVPWM_closeloop/SVPWM调制/SVPWM/第二大扇区羊角分配 ==
  data: n input; T1 input; T2 input; T3 input; t11 output; t21 output; t31 output
function [t11,t21,t31] = VectorShare(n,T1,T2,T3)
t11 = 0;
t21 = 0;
t31 = 0;
if (n==1)
    t11 = T1/2;
    t21 = T1/2+T3;
    t31 = -T1/2;
end
if (n==2)
    t11 = -T1/2;
    t21 = T1/2;
    t31 = -T1/2-T2;
end
if (n==3)
    t11 = T1/2;
    t21 = T1/2+T2+T3;
    t31 = -T1/2-T2;
end
if (n==4)
    t11 = -T1/2;
    t21 = T1/2+T3;
    t31 = -T1/2-T2-T3;
end
if (n==5)
    t11 = T1/2+T3;
    t21 = T1/2+T2+T3;
    t31 = -T1/2-T2-T3;
end
if (n==6)
    t11 = -T1/2-T2;
    t21 = T1/2+T2+T3;
    t31 = -T1/2-T2-T3;
end

== matlab function SVPWM_closeloop/SVPWM调制/SVPWM/羊角波生成 ==
  data: N input; t11 input; t12 input; t13 input; YJA output; YJB output; YJC output; t21 input; t22 input; t23 input
function [YJA,YJB,YJC] = YangJiao(N,t11,t12,t13,t21,t22,t23)
YJA = 0;
YJB = 0;
YJC = 0;
if (N==1)
    YJA = t11;
    YJB = t12;
    YJC = t13;
end
if (N==2)
    YJA = t21;
    YJB = t22;
    YJC = t23;
end
if (N==3)
    YJA = t13;
    YJB = t11;
    YJC = t12;
end
if (N==4)
    YJA = t23;
    YJB = t21;
    YJC = t22;
end
if (N==5)
    YJA = t12;
    YJB = t13;
    YJC = t11;
end
if (N==6)
    YJA = t22;
    YJB = t23;
    YJC = t21;
end

== matlab function SVPWM_closeloop/SVPWM调制/SVPWM/大扇区 ==
  data: u input; N output; theta output
function [N, theta] = BigVectorSwitch(u)

% Transfer to Section I
N = 0;
theta = 0;
thetaset = ceil(u/(pi/3));

u1 = u;
u2 = u-pi/3;
u3 = u-2*pi/3;
u4 = u-pi;
u5 = u-4*pi/3;
u6 = u-5*pi/3;

% Judge Section and Mapping
if (thetaset == 1)
    theta = u1;
    N = 4;
end

if (thetaset == 2)
    theta = u2;
    N = 5;
end

if (thetaset == 3)
    theta = u3;
    N = 6;
end

if (thetaset == 4)
    theta = u4;
    N = 1;
end

if (thetaset == 5)
    theta = u5;
    N = 2;
end

if (thetaset == 6)
    theta = u6;
    N = 3;
end

== matlab function SVPWM_closeloop/SVPWM调制/SVPWM/Reference Voltage ==
  data: ua input; Uref output; ub input; uc input
function Uref = volt(ua,ub,uc)

Uref = (2/3) * (ua + ub*exp(1i*2*pi/3) + uc*exp(-1i*2*pi/3));

== matlab function SVPWM_closeloop/SVPWM调制/SVPWM/小扇区 ==
  data: m input; n output; theta input
function n = SmallVectorSwitch(m, theta)

l_BD = -0.5 + m*sin(theta);
l_AB =  sqrt(3)*m*cos(theta) + m*sin(theta) -1;
l_AD = -sqrt(3)*m*cos(theta) + m*sin(theta) +1;

if (theta <= pi/6)
    if (l_AB <= 0)
        n=1;
    elseif (l_AD <= 0)
        n=5;
    else
        n=3;
    end
else
    if (l_AB <= 0)
        n=2;
    elseif (l_BD >= 0)
        n=6;
    else
        n=4;
    end
end

== matlab function SVPWM_closeloop/SVPWM调制/SVPWM/矢量作用时间 ==
  data: n input; m input; Ts input; TA output; theta input; TB output; TC output
function [TA,TB,TC] = VectorTime(n,m,Ts,theta)

TA=0;
TB=0;
TC=0;

if (n==1 || n==2)
    TA = 2*m*Ts*sin(theta);
    TB = Ts*(1-2*m*sin(theta+pi/3));
    TC = 2*m*Ts*sin(-theta+pi/3);
end

if (n==3 || n==4)
    TA = Ts*(1-2*m*sin(theta));
    TB = Ts*(2*m*sin(pi/3+theta)-1);
    TC = Ts*(1-2*m*sin(pi/3-theta));
end

if (n==5)
    TA = 2*m*Ts*sin(theta);
    TB = 2*Ts*(1-m*sin(pi/3 + theta));
    TC = Ts*(2*m*sin(pi/3-theta)-1);
end

if (n==6)
    TA = Ts*(2*m*sin(theta)-1);
    TB = 2*Ts*(1-m*sin(pi/3 + theta));
    TC = 2*m*Ts*sin(pi/3-theta);
end

== matlab function SVPWM_closeloop/SVPWM调制/SVPWM/上半周期时间分配 ==
  data: TA input; TB input; TC input; n input; t1 output; t2 output; t3 output
function [t1,t2,t3] = TimeShare(TA,TB,TC,n)

t1=0;
t2=0;
t3=0;

if (n==1)
    t1 = TC;
    t2 = TA;
    t3 = TB;
end

if (n==2)
    t1 = TA;
    t2 = TB;
    t3 = TC;
end

if (n==3)
    t1 = TA;
    t2 = TC;
    t3 = TB;
end

if (n==4)
    t1 = TC;
    t2 = TB;
    t3 = TA;
end

if (n==5)
    t1 = TB;
    t2 = TC;
    t3 = TA;
end

if (n==6)
    t1 = TB;
    t2 = TC;
    t3 = TA;
end

== matlab function SVPWM_closeloop/SVPWM调制/SVPWM/下半周期时间分配 ==
  data: TA input; TB input; TC input; n input; t1 output; t2 output; t3 output
function [t1,t2,t3] = TimeShare(TA,TB,TC,n)

t1=0;
t2=0;
t3=0;

if (n==1)
    t1 = TC;
    t2 = TB;
    t3 = TA;
end

if (n==2)
    t1 = TA;
    t2 = TC;
    t3 = TB;
end

if (n==3)
    t1 = TA;
    t2 = TB;
    t3 = TC;
end

if (n==4)
    t1 = TC;
    t2 = TA;
    t3 = TB;
end

if (n==5)
    t1 = TB;
    t2 = TA;
    t3 = TC;
end

if (n==6)
    t1 = TB;
    t2 = TA;
    t3 = TC;
end

== matlab function SVPWM_closeloop/SVPWM调制/SVPWM/按规律选择实际时间分配 ==
  data: ta1 input; tb1 input; tc1 input; ta2 input; T1 output; T2 output; T3 output; tb2 input; tc2 input; N input
function [T1,T2,T3] = SwitchTime(ta1,tb1,tc1,ta2,tb2,tc2,N)
T1 = 0;
T2 = 0;
T3 = 0;
if (N == 1)
    T1 = ta1;
    T2 = tb1;
    T3 = tc1;
end

if (N == 2)
    T1 = ta2;
    T2 = tb2;
    T3 = tc2;
end

if (N == 3)
    T1 = ta1;
    T2 = tb1;
    T3 = tc1;
end

if (N == 4)
    T1 = ta2;
    T2 = tb2;
    T3 = tc2;
end

if (N == 5)
    T1 = ta1;
    T2 = tb1;
    T3 = tc1;
end

if (N == 6)
    T1 = ta2;
    T2 = tb2;
    T3 = tc2;
end

== matlab function SVPWM_closeloop/SVPWM调制/SVPWM/第一大扇区羊角分配 ==
  data: n input; T1 input; T2 input; T3 input; t11 output; t21 output; t31 output
function [t11,t21,t31] = VectorShare(n,T1,T2,T3)
t11 = 0;
t21 = 0;
t31 = 0;
if (n==1)
    t11 = T1/2;
    t21 = -T1/2;
    t31 = -T1/2-T2;
end
if (n==2)
    t11 = T1/2+T3;
    t21 = T1/2;
    t31 = -T1/2;
end
if (n==3)
    t11 = T1/2+T3;
    t21 = -T1/2;
    t31 = -T1/2-T2-T3;
end
if (n==4)
    t11 = T1/2+T2+T3;
    t21 = T1/2;
    t31 = -T1/2-T2;
end
if (n==5)
    t11 = T1/2+T2+T3;
    t21 = -T1/2-T2;
    t31 = -T1/2-T2-T3;
end
if (n==6)
    t11 = T1/2+T2+T3;
    t21 = T1/2+T3;
    t31 = -T1/2-T2-T3;
end
